simulink model "seti_ct"  (Simulink 6.2)
settings: Solver=ode45  StartTime=0.0  StopTime=100000  RelTol=1e-3
values from neighbouring files (symbols this model uses):
  bigColBits = 0    [address_gen_dram_mask.m]
  bigRowBits = log2(bigRowLength)    [address_gen_dram_mask.m]
  smallColBits = 0    [address_gen_dram_mask.m]
  smallRowBits = log2(smallRowLength)    [address_gen_dram_mask.m]
libraries: xbsIndex_r3 x487, xps_library x45, casper_library x18, fft_library x1
(part 2 of 3)

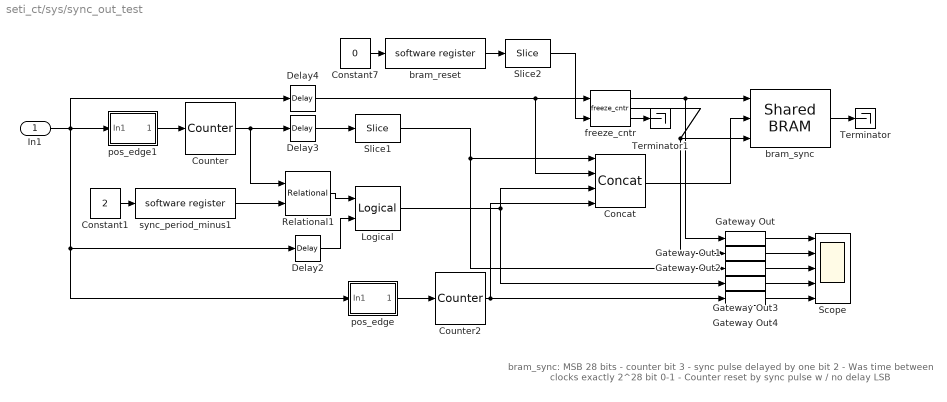
== system seti_ct/sys/sync_out_test ==
  note: bram_sync: MSB
      | 28 bits - counter
      | bit 3 - sync pulse delayed by one
      | bit 2 - Was time between clocks exactly 2^28
      | bit 0-1 - Counter reset by sync pulse w / no delay
      | LSB
  In1 : Inport  Port=1  LatchInput=off
  Concat : xbsIndex_r3/Concat  num_inputs=4  explicit_period=off  period=1  dbl_ovrd=off
  Constant1 : Constant  Value=2
  Constant7 : Constant  Value=0
  Counter : xbsIndex_r3/Counter  cnt_type=Free Running  n_bits=32  bin_pt=0  arith_type=Unsigned  start_count=0  cnt_to=2^4-1  cnt_by_val=1  operation=Up  explicit_period=on  period=1  load_pin=off  rst=on  en=off  dbl_ovrd=off  show_param=off  use_rpm=on  gen_core=off
      settings: xl_area=[0, 0, 0, 0, 0, 0, 0]
  Counter2 : xbsIndex_r3/Counter  cnt_type=Count Limited  n_bits=2  bin_pt=0  arith_type=Unsigned  start_count=0  cnt_to=3  cnt_by_val=1  operation=Up  explicit_period=on  period=1  load_pin=off  rst=on  en=off  dbl_ovrd=off  show_param=off  use_rpm=on  gen_core=off
      settings: xl_area=[0, 0, 0, 0, 0, 0, 0]
  Delay2 : xbsIndex_r3/Delay  latency=1  reg_retiming=off  explicit_period=on  period=1  en=off  accept_only_valid=off  init_zero=on  dbl_ovrd=off  show_param=off
      settings: xl_area=[0, 0, 0, 0, 0, 0, 0]
  Delay3 : xbsIndex_r3/Delay  latency=1  reg_retiming=off  explicit_period=on  period=1  en=off  accept_only_valid=off  init_zero=on  dbl_ovrd=off  show_param=off
      settings: xl_area=[0, 0, 0, 0, 0, 0, 0]
  Delay4 : xbsIndex_r3/Delay  latency=1  reg_retiming=off  explicit_period=on  period=1  en=off  accept_only_valid=off  init_zero=on  dbl_ovrd=off  show_param=off
      settings: xl_area=[0, 0, 0, 0, 0, 0, 0]
  Gateway Out{,1..4} (5 alike) : xbsIndex_r3/Gateway Out  output_type=Double  nbits=8  bin_pt=6  arith_type=Boolean  quantization=Truncate  overflow=Wrap  hdl_port=on  timing_constraint=None  locs_specified=off  LOCs={}  needs_fixed_name=off  show_param=off
      settings: xl_area=[0, 0, 0, 0, 0, 0, 0]
  Logical : xbsIndex_r3/Logical  logical_function=AND  inputs=2  precision=Full  arith_type=Unsigned  n_bits=2  bin_pt=0  align_bp=on  latency=0  explicit_period=off  period=1  en=off  dbl_ovrd=off  show_param=off
      settings: xl_area=[0, 0, 0, 0, 0, 0, 0]
  Relational1 : xbsIndex_r3/Relational  mode=a=b  latency=1  explicit_period=on  period=1  en=off  dbl_ovrd=off  show_param=off
      settings: xl_area=[0, 0, 0, 0, 0, 0, 0]
  Scope : Scope  NumInputPorts=5
      settings: YMin=-5~-5~-5~-5~-5  YMax=5~5~5~5~5
  Slice1 : xbsIndex_r3/Slice  mode=Lower Bit Location + Width  nbits=28  bit1=0  base1=MSB of Input  bit0=0  base0=LSB of Input  boolean_output=off  explicit_period=off  period=1  dbl_ovrd=off
  Slice2 : xbsIndex_r3/Slice  mode=Lower Bit Location + Width  nbits=1  bit1=0  base1=MSB of Input  bit0=0  base0=LSB of Input  boolean_output=on  explicit_period=off  period=1  dbl_ovrd=off
  Terminator : Terminator
  Terminator1 : Terminator
  bram_reset : xps_library/software register  Tag=xps:sw_reg  io_dir=From Processor  arith_type=Unsigned  bitwidth=32  bin_pt=0  sample_period=1  gw_name=seti_ct_sys_sync_out_test_bram_reset_user_data_out
  bram_sync : xps_library/Shared BRAM  Tag=xps:bram  arith_type=Unsigned  addr_width=12  data_width=32  data_bin_pt=0  init_vals=0  sample_rate=1
  freeze_cntr : casper_library/Misc/freeze_cntr  CounterBits=12
  pos_edge : Subsystem
  pos_edge1 : Subsystem
  sync_period_minus1 : xps_library/software register  Tag=xps:sw_reg  io_dir=From Processor  arith_type=Unsigned  bitwidth=32  bin_pt=0  sample_period=1  gw_name=seti_ct_sys_sync_out_test_sync_period_minus1_user_data_out
  wires:
  Counter/1 -> Relational1/1, Delay3/1
  Relational1/1 -> Logical/1
  Delay2/1 -> Logical/2
  Constant1/1 -> sync_period_minus1/1
  sync_period_minus1/1 -> Relational1/2
  freeze_cntr/1 -> bram_sync/1, Gateway Out/1
  freeze_cntr/2 -> bram_sync/3, Gateway Out1/1
  Delay3/1 -> Slice1/1
  Delay4/1 -> Concat/2, freeze_cntr/1
  Constant7/1 -> bram_reset/1
  bram_reset/1 -> Slice2/1
  Gateway Out/1 -> Scope/1
  Gateway Out1/1 -> Scope/2
  Gateway Out2/1 -> Scope/3
  Gateway Out3/1 -> Scope/4
  Concat/1 -> bram_sync/2
  Logical/1 -> Gateway Out3/1, Concat/3
  Slice2/1 -> freeze_cntr/2
  Gateway Out4/1 -> Scope/5
  pos_edge/1(Out1) -> Counter2/1
  Counter2/1 -> Gateway Out4/1, Concat/4
  pos_edge1/1(Out1) -> Counter/1
  Slice1/1 -> Concat/1, Gateway Out2/1
  In1/1 -> pos_edge1/1(In1), Delay4/1, Delay2/1, pos_edge/1(In1)
  bram_sync/1 -> Terminator/1
  freeze_cntr/3 -> Terminator1/1

== system seti_ct/sys/trig_delay ==
  data_in : Inport  Port=1  LatchInput=off
  trig_in : Inport  Port=2  LatchInput=off
  delay : Inport  Port=3  LatchInput=off
  Constant : xbsIndex_r3/Constant  const=1  equ=P=C  arith_type=Boolean  n_bits=32  bin_pt=0  opselect=C  inp2=PCIN>>17  opr=+  inp1=P  carry=CIN  iostate=0  explicit_period=on  period=1  dbl_ovrd=off
  Counter : xbsIndex_r3/Counter  cnt_type=Free Running  n_bits=32  bin_pt=0  arith_type=Unsigned  start_count=0  cnt_to=Inf  cnt_by_val=1  operation=Up  explicit_period=on  period=1  load_pin=off  rst=on  en=on  dbl_ovrd=off  show_param=off  use_rpm=on  gen_core=off
      settings: xl_area=[0, 0, 0, 0, 0, 0, 0]
  Delay : xbsIndex_r3/Delay  latency=2  reg_retiming=off  explicit_period=on  period=1  en=off  accept_only_valid=off  init_zero=on  dbl_ovrd=off  show_param=off
      settings: xl_area=[0, 0, 0, 0, 0, 0, 0]
  Gateway Out : xbsIndex_r3/Gateway Out  output_type=Double  nbits=8  bin_pt=6  arith_type=Boolean  quantization=Truncate  overflow=Wrap  hdl_port=on  timing_constraint=None  locs_specified=off  LOCs={}  needs_fixed_name=off  show_param=off
      settings: xl_area=[0, 0, 0, 0, 0, 0, 0]
  Gateway Out1 : xbsIndex_r3/Gateway Out  output_type=Double  nbits=8  bin_pt=6  arith_type=Boolean  quantization=Truncate  overflow=Wrap  hdl_port=on  timing_constraint=None  locs_specified=off  LOCs={}  needs_fixed_name=off  show_param=off
      settings: xl_area=[0, 0, 0, 0, 0, 0, 0]
  Register : xbsIndex_r3/Register  init=0  reg_only_valid=off  explicit_period=on  period=1  rst=on  en=on  out_en=off  dbl_ovrd=off  show_param=off
      settings: xl_area=[0, 0, 0, 0, 0, 0, 0]
  Relational : xbsIndex_r3/Relational  mode=a=b  latency=1  explicit_period=on  period=1  en=on  dbl_ovrd=off  show_param=off
      settings: xl_area=[0, 0, 0, 0, 0, 0, 0]
  Scope : Scope  NumInputPorts=2
      settings: YMin=-5~-5  YMax=5~5
  posedge : casper_library/Misc/posedge  Tag=Rising Edge Detector
  data_out : Outport
  trig_out : Outport  Port=2
  wires:
  delay/1 -> Relational/1
  trig_in/1 -> Register/3, Gateway Out1/1
  Constant/1 -> Register/1
  Relational/1 -> Register/2, Counter/1, Gateway Out/1, posedge/1
  Register/1 -> Counter/2, Relational/3
  Counter/1 -> Relational/2
  Gateway Out/1 -> Scope/1
  Gateway Out1/1 -> Scope/2
  data_in/1 -> Delay/1
  Delay/1 -> data_out/1
  posedge/1 -> trig_out/1

== system seti_ct/sys/trig_delay1 ==
  data_in : Inport  Port=1  LatchInput=off
  trig_in : Inport  Port=2  LatchInput=off
  delay : Inport  Port=3  LatchInput=off
  Constant : xbsIndex_r3/Constant  const=1  equ=P=C  arith_type=Boolean  n_bits=32  bin_pt=0  opselect=C  inp2=PCIN>>17  opr=+  inp1=P  carry=CIN  iostate=0  explicit_period=on  period=1  dbl_ovrd=off
  Counter : xbsIndex_r3/Counter  cnt_type=Free Running  n_bits=32  bin_pt=0  arith_type=Unsigned  start_count=0  cnt_to=Inf  cnt_by_val=1  operation=Up  explicit_period=on  period=1  load_pin=off  rst=on  en=on  dbl_ovrd=off  show_param=off  use_rpm=on  gen_core=off
      settings: xl_area=[0, 0, 0, 0, 0, 0, 0]
  Delay : xbsIndex_r3/Delay  latency=2  reg_retiming=off  explicit_period=on  period=1  en=off  accept_only_valid=off  init_zero=on  dbl_ovrd=off  show_param=off
      settings: xl_area=[0, 0, 0, 0, 0, 0, 0]
  Gateway Out : xbsIndex_r3/Gateway Out  output_type=Double  nbits=8  bin_pt=6  arith_type=Boolean  quantization=Truncate  overflow=Wrap  hdl_port=on  timing_constraint=None  locs_specified=off  LOCs={}  needs_fixed_name=off  show_param=off
      settings: xl_area=[0, 0, 0, 0, 0, 0, 0]
  Gateway Out1 : xbsIndex_r3/Gateway Out  output_type=Double  nbits=8  bin_pt=6  arith_type=Boolean  quantization=Truncate  overflow=Wrap  hdl_port=on  timing_constraint=None  locs_specified=off  LOCs={}  needs_fixed_name=off  show_param=off
      settings: xl_area=[0, 0, 0, 0, 0, 0, 0]
  Register : xbsIndex_r3/Register  init=0  reg_only_valid=off  explicit_period=on  period=1  rst=on  en=on  out_en=off  dbl_ovrd=off  show_param=off
      settings: xl_area=[0, 0, 0, 0, 0, 0, 0]
  Relational : xbsIndex_r3/Relational  mode=a=b  latency=1  explicit_period=on  period=1  en=on  dbl_ovrd=off  show_param=off
      settings: xl_area=[0, 0, 0, 0, 0, 0, 0]
  Scope : Scope  NumInputPorts=2
      settings: YMin=-5~-5  YMax=5~5
  posedge : casper_library/Misc/posedge  Tag=Rising Edge Detector
  data_out : Outport
  trig_out : Outport  Port=2
  wires:
  delay/1 -> Relational/1
  trig_in/1 -> Register/3, Gateway Out1/1
  Constant/1 -> Register/1
  Relational/1 -> Register/2, Counter/1, Gateway Out/1, posedge/1
  Register/1 -> Counter/2, Relational/3
  Counter/1 -> Relational/2
  Gateway Out/1 -> Scope/1
  Gateway Out1/1 -> Scope/2
  data_in/1 -> Delay/1
  Delay/1 -> data_out/1
  posedge/1 -> trig_out/1

== system seti_ct/sys/trig_delay2 ==
  data_in : Inport  Port=1  LatchInput=off
  trig_in : Inport  Port=2  LatchInput=off
  delay : Inport  Port=3  LatchInput=off
  Constant : xbsIndex_r3/Constant  const=1  equ=P=C  arith_type=Boolean  n_bits=32  bin_pt=0  opselect=C  inp2=PCIN>>17  opr=+  inp1=P  carry=CIN  iostate=0  explicit_period=on  period=1  dbl_ovrd=off
  Counter : xbsIndex_r3/Counter  cnt_type=Free Running  n_bits=32  bin_pt=0  arith_type=Unsigned  start_count=0  cnt_to=Inf  cnt_by_val=1  operation=Up  explicit_period=on  period=1  load_pin=off  rst=on  en=on  dbl_ovrd=off  show_param=off  use_rpm=on  gen_core=off
      settings: xl_area=[0, 0, 0, 0, 0, 0, 0]
  Delay : xbsIndex_r3/Delay  latency=2  reg_retiming=off  explicit_period=on  period=1  en=off  accept_only_valid=off  init_zero=on  dbl_ovrd=off  show_param=off
      settings: xl_area=[0, 0, 0, 0, 0, 0, 0]
  Gateway Out : xbsIndex_r3/Gateway Out  output_type=Double  nbits=8  bin_pt=6  arith_type=Boolean  quantization=Truncate  overflow=Wrap  hdl_port=on  timing_constraint=None  locs_specified=off  LOCs={}  needs_fixed_name=off  show_param=off
      settings: xl_area=[0, 0, 0, 0, 0, 0, 0]
  Gateway Out1 : xbsIndex_r3/Gateway Out  output_type=Double  nbits=8  bin_pt=6  arith_type=Boolean  quantization=Truncate  overflow=Wrap  hdl_port=on  timing_constraint=None  locs_specified=off  LOCs={}  needs_fixed_name=off  show_param=off
      settings: xl_area=[0, 0, 0, 0, 0, 0, 0]
  Register : xbsIndex_r3/Register  init=0  reg_only_valid=off  explicit_period=on  period=1  rst=on  en=on  out_en=off  dbl_ovrd=off  show_param=off
      settings: xl_area=[0, 0, 0, 0, 0, 0, 0]
  Relational : xbsIndex_r3/Relational  mode=a=b  latency=1  explicit_period=on  period=1  en=on  dbl_ovrd=off  show_param=off
      settings: xl_area=[0, 0, 0, 0, 0, 0, 0]
  Scope : Scope  NumInputPorts=2
      settings: YMin=-5~-5  YMax=5~5
  posedge : casper_library/Misc/posedge  Tag=Rising Edge Detector
  data_out : Outport
  trig_out : Outport  Port=2
  wires:
  delay/1 -> Relational/1
  trig_in/1 -> Register/3, Gateway Out1/1
  Constant/1 -> Register/1
  Relational/1 -> Register/2, Counter/1, Gateway Out/1, posedge/1
  Register/1 -> Counter/2, Relational/3
  Counter/1 -> Relational/2
  Gateway Out/1 -> Scope/1
  Gateway Out1/1 -> Scope/2
  data_in/1 -> Delay/1
  Delay/1 -> data_out/1
  posedge/1 -> trig_out/1

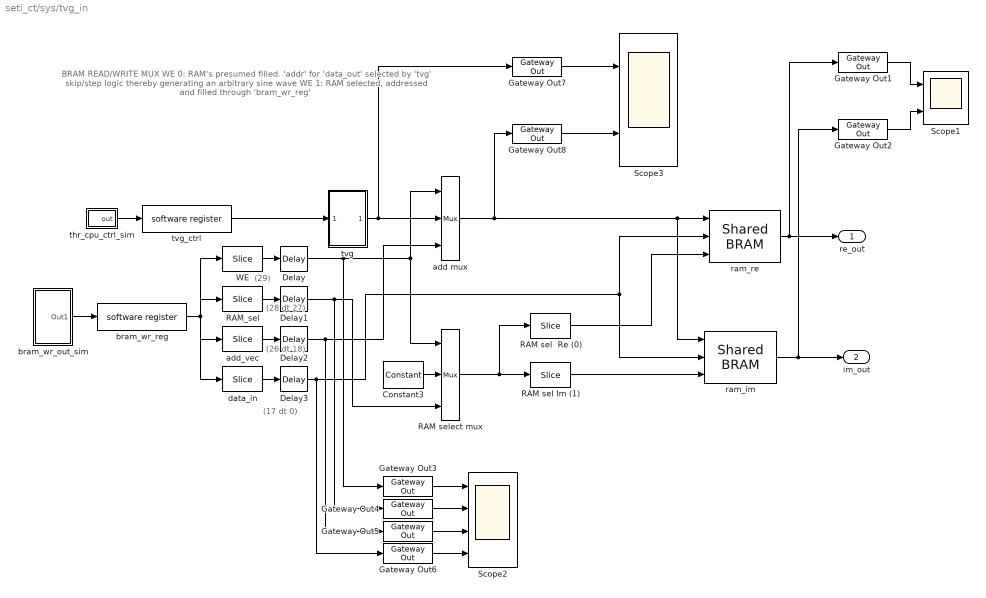
== system seti_ct/sys/tvg_in ==
  note: BRAM READ/WRITE MUX
      | WE 0: RAM's presumed filled.
      | 'addr' for 'data_out' selected
      | by 'tvg' skip/step logic thereby
      | generating an arbitrary sine wave
      | WE 1: RAM selected, addressed
      | and filled through
      | 'bram_wr_reg'
  note: (29)
  note: (28 dt 27)
  note: (17 dt 0)
  note: (26 dt 18)
  Constant3 : xbsIndex_r3/Constant  const=0  equ=P=C  arith_type=Unsigned  n_bits=4  bin_pt=0  opselect=C  inp2=PCIN>>17  opr=+  inp1=P  carry=CIN  iostate=0  explicit_period=on  period=1  dbl_ovrd=off
  Delay{,1..3} (4 alike) : xbsIndex_r3/Delay  latency=1  reg_retiming=off  explicit_period=on  period=1  en=off  accept_only_valid=off  init_zero=on  dbl_ovrd=off  show_param=off
      settings: xl_area=[0, 0, 0, 0, 0, 0, 0]
  Gateway Out{1..8} (8 alike) : xbsIndex_r3/Gateway Out  output_type=Double  nbits=8  bin_pt=6  arith_type=Boolean  quantization=Truncate  overflow=Wrap  hdl_port=on  timing_constraint=None  locs_specified=off  LOCs={}  needs_fixed_name=off  show_param=off
      settings: xl_area=[0, 0, 0, 0, 0, 0, 0]
  RAM sel  Re (0) : xbsIndex_r3/Slice  mode=Lower Bit Location + Width  nbits=1  bit1=0  base1=MSB of Input  bit0=0  base0=LSB of Input  boolean_output=on  explicit_period=on  period=1  dbl_ovrd=off
  RAM sel Im (1) : xbsIndex_r3/Slice  mode=Lower Bit Location + Width  nbits=1  bit1=0  base1=MSB of Input  bit0=1  base0=LSB of Input  boolean_output=on  explicit_period=on  period=1  dbl_ovrd=off
  RAM select mux : xbsIndex_r3/Mux  inputs=2  precision=Full  arith_type="Signed  (2's comp)"  n_bits=8  bin_pt=2  quantization=Truncate  overflow=Wrap  latency=0  explicit_period=on  period=1  en=off  dbl_ovrd=off  show_param=off  mux_type=off  use_rpm=off  gen_core=off
      settings: xl_area=[0, 0, 0, 0, 0, 0, 0]
  RAM_sel : xbsIndex_r3/Slice  mode=Lower Bit Location + Width  nbits=2  bit1=10  base1=MSB of Input  bit0=27  base0=LSB of Input  boolean_output=off  explicit_period=on  period=1  dbl_ovrd=off
  Scope1 : Scope  NumInputPorts=2
      settings: YMin=-5~-5  YMax=5~5  SaveName=ScopeData2
  Scope2 : Scope  NumInputPorts=4
      settings: YMin=-5~-5~-5~-5  YMax=5~5~5~5
  Scope3 : Scope  NumInputPorts=2
      settings: YMin=-5~-5  YMax=5~5  SaveName=ScopeData3
  WE : xbsIndex_r3/Slice  mode=Lower Bit Location + Width  nbits=1  bit1=10  base1=MSB of Input  bit0=29  base0=LSB of Input  boolean_output=off  explicit_period=on  period=1  dbl_ovrd=off
  add mux : xbsIndex_r3/Mux  inputs=2  precision=Full  arith_type="Signed  (2's comp)"  n_bits=8  bin_pt=2  quantization=Truncate  overflow=Wrap  latency=0  explicit_period=on  period=1  en=off  dbl_ovrd=off  show_param=off  mux_type=off  use_rpm=off  gen_core=off
      settings: xl_area=[0, 0, 0, 0, 0, 0, 0]
  add_vec : xbsIndex_r3/Slice  mode=Lower Bit Location + Width  nbits=9  bit1=0  base1=MSB of Input  bit0=18  base0=LSB of Input  boolean_output=off  explicit_period=on  period=1  dbl_ovrd=off
  bram_wr_out_sim : Subsystem  mask{we_enable=0, ram_sel=3, add_vec=512, data_in=32}
      mask prompts: we_enable "Write enable"; ram_sel "RAM selector (1 = Re; 2 = Im; 3 = both)"; add_vec "RAM address"; data_in "Data in"
  bram_wr_reg : xps_library/software register  Tag=xps:sw_reg  io_dir=From Processor  arith_type=Unsigned  bitwidth=32  bin_pt=0  sample_period=1  gw_name=seti_ct_sys_tvg_in_bram_wr_reg_user_data_out
  data_in : xbsIndex_r3/Slice  mode=Lower Bit Location + Width  nbits=18  bit1=0  base1=MSB of Input  bit0=0  base0=LSB of Input  boolean_output=off  explicit_period=on  period=1  dbl_ovrd=off
  ram_im : xps_library/Shared BRAM  Tag=xps:bram  arith_type="Signed  (2's comp)"  addr_width=11  data_width=32  data_bin_pt=0  init_vals=[1:2^11]  sample_rate=1
  ram_re : xps_library/Shared BRAM  Tag=xps:bram  arith_type="Signed  (2's comp)"  addr_width=11  data_width=32  data_bin_pt=0  init_vals=[1:2^11]  sample_rate=1
  thr_cpu_ctrl_sim : Subsystem  mask{tvg_skip=1, tvg_stall=2, tvg_length=5}
      mask prompts: tvg_skip "Skip"; tvg_stall "Stall"; tvg_length "Length"
      mask help:
      | Mux Data for CT and FFT Syncs:
      |
      | 0 -> Interchip Connection
      | 1 -> User Generated External Sync
      | 2 -> Periodic Sync Generator
      | 3 -> Periodic Sync Generator (Same as 2)
      |
      | Mux Data for CT and FFT Inputs:
      |
      | 0 -> Interchip Connection
      | 1 -> Test Vector Generator (TVG)
      | 2 -> All Zeroes (0's)
      | 3 -> All Ones (1's)
  tvg : Subsystem  mask(Test Vector Generator(TVG)){tvg_skip=1, tvg_stall=1, tvg_length=512}
      mask prompts: tvg_skip "Skip"; tvg_stall "Stall"; tvg_length "Length"
  tvg_ctrl : xps_library/software register  Tag=xps:sw_reg  io_dir=From Processor  arith_type=Unsigned  bitwidth=32  bin_pt=0  sample_period=1  gw_name=seti_ct_sys_tvg_in_tvg_ctrl_user_data_out
  re_out : Outport
  im_out : Outport  Port=2
  wires:
  tvg_ctrl/1 -> tvg/1(In1)
  tvg/1(Out1) -> add mux/2, Gateway Out7/1
  Constant3/1 -> RAM select mux/2
  RAM select mux/1 -> RAM sel  Re (0)/1, RAM sel Im (1)/1
  RAM sel  Re (0)/1 -> ram_re/3
  WE/1 -> Delay/1
  Gateway Out1/1 -> Scope1/1
  Gateway Out2/1 -> Scope1/2
  thr_cpu_ctrl_sim/1(out) -> tvg_ctrl/1
  bram_wr_reg/1 -> data_in/1, add_vec/1, RAM_sel/1, WE/1
  add_vec/1 -> Delay2/1
  RAM_sel/1 -> Delay1/1
  add mux/1 -> ram_im/1, ram_re/1, Gateway Out8/1
  data_in/1 -> Delay3/1
  RAM sel Im (1)/1 -> ram_im/3
  ram_re/1 -> Gateway Out1/1, re_out/1
  ram_im/1 -> Gateway Out2/1, im_out/1
  bram_wr_out_sim/1(Out1) -> bram_wr_reg/1
  Gateway Out3/1 -> Scope2/1
  Gateway Out4/1 -> Scope2/2
  Gateway Out5/1 -> Scope2/3
  Gateway Out6/1 -> Scope2/4
  Delay/1 -> Gateway Out3/1, add mux/1, RAM select mux/1
  Delay1/1 -> Gateway Out4/1, RAM select mux/3
  Delay2/1 -> Gateway Out5/1, add mux/3
  Delay3/1 -> Gateway Out6/1, ram_re/2, ram_im/2
  Gateway Out7/1 -> Scope3/1
  Gateway Out8/1 -> Scope3/2

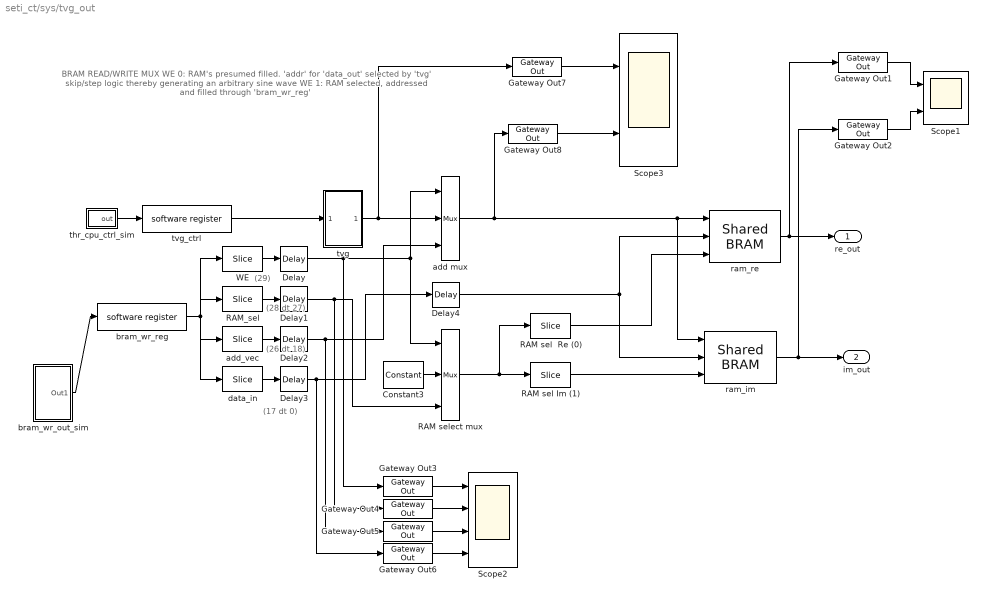
== system seti_ct/sys/tvg_out ==
  note: BRAM READ/WRITE MUX
      | WE 0: RAM's presumed filled.
      | 'addr' for 'data_out' selected
      | by 'tvg' skip/step logic thereby
      | generating an arbitrary sine wave
      | WE 1: RAM selected, addressed
      | and filled through
      | 'bram_wr_reg'
  note: (29)
  note: (28 dt 27)
  note: (17 dt 0)
  note: (26 dt 18)
  Constant3 : xbsIndex_r3/Constant  const=0  equ=P=C  arith_type=Unsigned  n_bits=4  bin_pt=0  opselect=C  inp2=PCIN>>17  opr=+  inp1=P  carry=CIN  iostate=0  explicit_period=on  period=1  dbl_ovrd=off
  Delay{,1..4} (5 alike) : xbsIndex_r3/Delay  latency=1  reg_retiming=off  explicit_period=on  period=1  en=off  accept_only_valid=off  init_zero=on  dbl_ovrd=off  show_param=off
      settings: xl_area=[0, 0, 0, 0, 0, 0, 0]
  Gateway Out{1..8} (8 alike) : xbsIndex_r3/Gateway Out  output_type=Double  nbits=8  bin_pt=6  arith_type=Boolean  quantization=Truncate  overflow=Wrap  hdl_port=on  timing_constraint=None  locs_specified=off  LOCs={}  needs_fixed_name=off  show_param=off
      settings: xl_area=[0, 0, 0, 0, 0, 0, 0]
  RAM sel  Re (0) : xbsIndex_r3/Slice  mode=Lower Bit Location + Width  nbits=1  bit1=0  base1=MSB of Input  bit0=0  base0=LSB of Input  boolean_output=on  explicit_period=on  period=1  dbl_ovrd=off
  RAM sel Im (1) : xbsIndex_r3/Slice  mode=Lower Bit Location + Width  nbits=1  bit1=0  base1=MSB of Input  bit0=1  base0=LSB of Input  boolean_output=on  explicit_period=on  period=1  dbl_ovrd=off
  RAM select mux : xbsIndex_r3/Mux  inputs=2  precision=Full  arith_type="Signed  (2's comp)"  n_bits=8  bin_pt=2  quantization=Truncate  overflow=Wrap  latency=1  explicit_period=on  period=1  en=off  dbl_ovrd=off  show_param=off  mux_type=off  use_rpm=off  gen_core=off
      settings: xl_area=[0, 0, 0, 0, 0, 0, 0]
  RAM_sel : xbsIndex_r3/Slice  mode=Lower Bit Location + Width  nbits=2  bit1=10  base1=MSB of Input  bit0=27  base0=LSB of Input  boolean_output=off  explicit_period=on  period=1  dbl_ovrd=off
  Scope1 : Scope  NumInputPorts=2
      settings: YMin=-5~-5  YMax=5~5  SaveName=ScopeData2
  Scope2 : Scope  NumInputPorts=4
      settings: YMin=-5~-5~-5~-5  YMax=5~5~5~5
  Scope3 : Scope  NumInputPorts=2
      settings: YMin=-5~-5  YMax=5~5  SaveName=ScopeData3
  WE : xbsIndex_r3/Slice  mode=Lower Bit Location + Width  nbits=1  bit1=10  base1=MSB of Input  bit0=29  base0=LSB of Input  boolean_output=off  explicit_period=on  period=1  dbl_ovrd=off
  add mux : xbsIndex_r3/Mux  inputs=2  precision=Full  arith_type="Signed  (2's comp)"  n_bits=8  bin_pt=2  quantization=Truncate  overflow=Wrap  latency=1  explicit_period=on  period=1  en=off  dbl_ovrd=off  show_param=off  mux_type=off  use_rpm=off  gen_core=off
      settings: xl_area=[0, 0, 0, 0, 0, 0, 0]
  add_vec : xbsIndex_r3/Slice  mode=Lower Bit Location + Width  nbits=9  bit1=0  base1=MSB of Input  bit0=18  base0=LSB of Input  boolean_output=off  explicit_period=on  period=1  dbl_ovrd=off
  bram_wr_out_sim : Subsystem  mask{we_enable=0, ram_sel=3, add_vec=512, data_in=32}
      mask prompts: we_enable "Write enable"; ram_sel "RAM selector (1 = Re; 2 = Im; 3 = both)"; add_vec "RAM address"; data_in "Data in"
  bram_wr_reg : xps_library/software register  Tag=xps:sw_reg  io_dir=From Processor  arith_type=Unsigned  bitwidth=32  bin_pt=0  sample_period=1  gw_name=seti_ct_sys_tvg_out_bram_wr_reg_user_data_out
  data_in : xbsIndex_r3/Slice  mode=Lower Bit Location + Width  nbits=18  bit1=0  base1=MSB of Input  bit0=0  base0=LSB of Input  boolean_output=off  explicit_period=on  period=1  dbl_ovrd=off
  ram_im : xps_library/Shared BRAM  Tag=xps:bram  arith_type="Signed  (2's comp)"  addr_width=11  data_width=32  data_bin_pt=0  init_vals=[1:2^11]  sample_rate=1
  ram_re : xps_library/Shared BRAM  Tag=xps:bram  arith_type="Signed  (2's comp)"  addr_width=11  data_width=32  data_bin_pt=0  init_vals=[1:2^11]  sample_rate=1
  thr_cpu_ctrl_sim : Subsystem  mask{tvg_skip=1, tvg_stall=2, tvg_length=5}
      mask prompts: tvg_skip "Skip"; tvg_stall "Stall"; tvg_length "Length"
      mask help:
      | Mux Data for CT and FFT Syncs:
      |
      | 0 -> Interchip Connection
      | 1 -> User Generated External Sync
      | 2 -> Periodic Sync Generator
      | 3 -> Periodic Sync Generator (Same as 2)
      |
      | Mux Data for CT and FFT Inputs:
      |
      | 0 -> Interchip Connection
      | 1 -> Test Vector Generator (TVG)
      | 2 -> All Zeroes (0's)
      | 3 -> All Ones (1's)
  tvg : Subsystem  mask(Test Vector Generator(TVG)){tvg_skip=1, tvg_stall=1, tvg_length=512}
      mask prompts: tvg_skip "Skip"; tvg_stall "Stall"; tvg_length "Length"
  tvg_ctrl : xps_library/software register  Tag=xps:sw_reg  io_dir=From Processor  arith_type=Unsigned  bitwidth=32  bin_pt=0  sample_period=1  gw_name=seti_ct_sys_tvg_out_tvg_ctrl_user_data_out
  re_out : Outport
  im_out : Outport  Port=2
  wires:
  tvg_ctrl/1 -> tvg/1(In1)
  tvg/1(Out1) -> add mux/2, Gateway Out7/1
  Constant3/1 -> RAM select mux/2
  RAM select mux/1 -> RAM sel  Re (0)/1, RAM sel Im (1)/1
  RAM sel  Re (0)/1 -> ram_re/3
  WE/1 -> Delay/1
  Gateway Out1/1 -> Scope1/1
  Gateway Out2/1 -> Scope1/2
  thr_cpu_ctrl_sim/1(out) -> tvg_ctrl/1
  bram_wr_reg/1 -> data_in/1, add_vec/1, RAM_sel/1, WE/1
  add_vec/1 -> Delay2/1
  RAM_sel/1 -> Delay1/1
  add mux/1 -> ram_im/1, ram_re/1, Gateway Out8/1
  data_in/1 -> Delay3/1
  RAM sel Im (1)/1 -> ram_im/3
  ram_re/1 -> Gateway Out1/1, re_out/1
  ram_im/1 -> Gateway Out2/1, im_out/1
  bram_wr_out_sim/1(Out1) -> bram_wr_reg/1
  Gateway Out3/1 -> Scope2/1
  Gateway Out4/1 -> Scope2/2
  Gateway Out5/1 -> Scope2/3
  Gateway Out6/1 -> Scope2/4
  Delay/1 -> Gateway Out3/1, add mux/1, RAM select mux/1
  Delay1/1 -> Gateway Out4/1, RAM select mux/3
  Delay2/1 -> Gateway Out5/1, add mux/3
  Delay3/1 -> Gateway Out6/1, Delay4/1
  Gateway Out7/1 -> Scope3/1
  Gateway Out8/1 -> Scope3/2
  Delay4/1 -> ram_re/2, ram_im/2

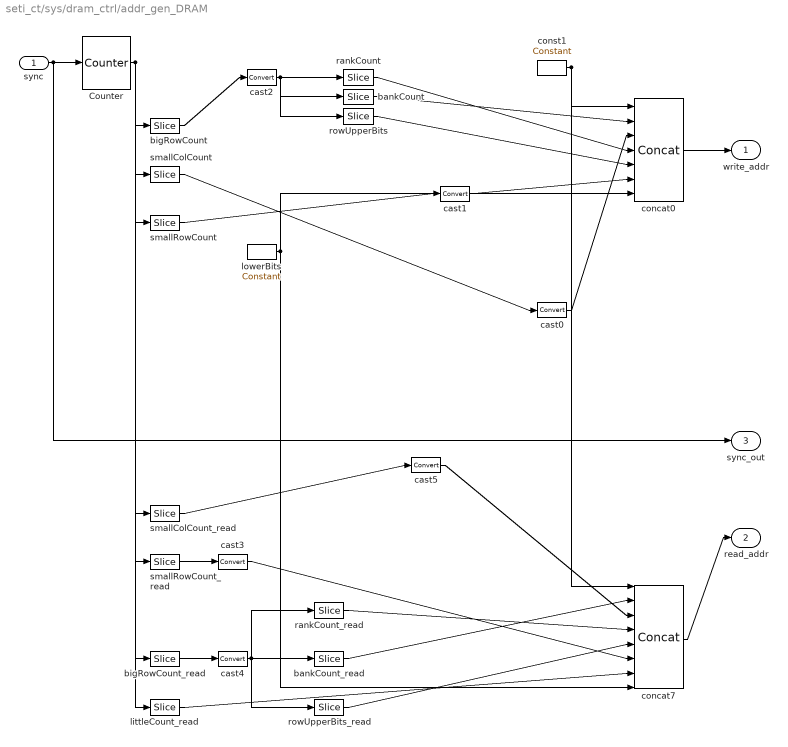
== system seti_ct/sys/dram_ctrl/addr_gen_DRAM ==
  sync : Inport  Port=1  LatchInput=off
  Counter : xbsIndex_r3/Counter  cnt_type=Free Running  n_bits=counterBitwidth  bin_pt=0  arith_type=Unsigned  start_count=0  cnt_to=Inf  cnt_by_val=1  operation=Up  explicit_period=off  period=1  load_pin=off  rst=on  en=off  dbl_ovrd=off  show_param=off  use_rpm=on  gen_core=off
      settings: xl_area=[0, 0, 0, 0, 0, 0, 0]
  bankCount : xbsIndex_r3/Slice  mode=Upper Bit Location + Width  nbits=2  bit1=-1  base1=MSB of Input  bit0=0  base0=LSB of Input  boolean_output=off  explicit_period=off  period=1  dbl_ovrd=off
  bankCount_read : xbsIndex_r3/Slice  mode=Upper Bit Location + Width  nbits=2  bit1=-1  base1=MSB of Input  bit0=0  base0=LSB of Input  boolean_output=off  explicit_period=off  period=1  dbl_ovrd=off
  bigRowCount : xbsIndex_r3/Slice  mode=Lower Bit Location + Width  nbits=bigRowBits  bit1=0  base1=MSB of Input  bit0=smallRowBits+smallColBits  base0=LSB of Input  boolean_output=off  explicit_period=off  period=1  dbl_ovrd=off
  bigRowCount_read : xbsIndex_r3/Slice  mode=Lower Bit Location + Width  nbits=bigRowBits  bit1=0  base1=MSB of Input  bit0=2  base0=LSB of Input  boolean_output=off  explicit_period=off  period=1  dbl_ovrd=off
  cast0 : xbsIndex_r3/Convert  arith_type=Unsigned  n_bits=14  bin_pt=0  quantization=Truncate  overflow=Wrap  latency=0  explicit_period=off  period=1  dbl_ovrd=off  show_param=off  inserted_by_tool=off  pipeline=off
      settings: xl_area=[0, 0, 0, 0, 0, 0, 0]
  cast1 : xbsIndex_r3/Convert  arith_type=Unsigned  n_bits=6  bin_pt=0  quantization=Truncate  overflow=Wrap  latency=0  explicit_period=off  period=1  dbl_ovrd=off  show_param=off  inserted_by_tool=off  pipeline=off
      settings: xl_area=[0, 0, 0, 0, 0, 0, 0]
  cast2 : xbsIndex_r3/Convert  arith_type=Unsigned  n_bits=7  bin_pt=0  quantization=Truncate  overflow=Wrap  latency=0  explicit_period=off  period=1  dbl_ovrd=off  show_param=off  inserted_by_tool=off  pipeline=off
      settings: xl_area=[0, 0, 0, 0, 0, 0, 0]
  cast3 : xbsIndex_r3/Convert  arith_type=Unsigned  n_bits=4  bin_pt=0  quantization=Truncate  overflow=Wrap  latency=0  explicit_period=off  period=1  dbl_ovrd=off  show_param=off  inserted_by_tool=off  pipeline=off
      settings: xl_area=[0, 0, 0, 0, 0, 0, 0]
  cast4 : xbsIndex_r3/Convert  arith_type=Unsigned  n_bits=7  bin_pt=0  quantization=Truncate  overflow=Wrap  latency=0  explicit_period=off  period=1  dbl_ovrd=off  show_param=off  inserted_by_tool=off  pipeline=off
      settings: xl_area=[0, 0, 0, 0, 0, 0, 0]
  cast5 : xbsIndex_r3/Convert  arith_type=Unsigned  n_bits=14  bin_pt=0  quantization=Truncate  overflow=Wrap  latency=0  explicit_period=off  period=1  dbl_ovrd=off  show_param=off  inserted_by_tool=off  pipeline=off
      settings: xl_area=[0, 0, 0, 0, 0, 0, 0]
  concat0 : xbsIndex_r3/Concat  num_inputs=7  explicit_period=off  period=1  dbl_ovrd=off
  concat7 : xbsIndex_r3/Concat  num_inputs=8  explicit_period=off  period=1  dbl_ovrd=off
  const1 : xbsIndex_r3/Constant  const=0  equ=P=C  arith_type=Unsigned  n_bits=2  bin_pt=0  opselect=C  inp2=PCIN>>17  opr=+  inp1=P  carry=CIN  iostate=0  explicit_period=on  period=1  dbl_ovrd=off
  littleCount_read : xbsIndex_r3/Slice  mode=Lower Bit Location + Width  nbits=2  bit1=0  base1=MSB of Input  bit0=0  base0=LSB of Input  boolean_output=off  explicit_period=off  period=1  dbl_ovrd=off
  lowerBits : xbsIndex_r3/Constant  const=0  equ=P=C  arith_type=Unsigned  n_bits=3  bin_pt=0  opselect=C  inp2=PCIN>>17  opr=+  inp1=P  carry=CIN  iostate=0  explicit_period=on  period=1  dbl_ovrd=off
  rankCount : xbsIndex_r3/Slice  mode=Upper Bit Location + Width  nbits=1  bit1=0  base1=MSB of Input  bit0=0  base0=LSB of Input  boolean_output=off  explicit_period=off  period=1  dbl_ovrd=off
  rankCount_read : xbsIndex_r3/Slice  mode=Upper Bit Location + Width  nbits=1  bit1=0  base1=MSB of Input  bit0=0  base0=LSB of Input  boolean_output=off  explicit_period=off  period=1  dbl_ovrd=off
  rowUpperBits : xbsIndex_r3/Slice  mode=Lower Bit Location + Width  nbits=4  bit1=0  base1=MSB of Input  bit0=0  base0=LSB of Input  boolean_output=off  explicit_period=off  period=1  dbl_ovrd=off
  rowUpperBits_read : xbsIndex_r3/Slice  mode=Lower Bit Location + Width  nbits=4  bit1=0  base1=MSB of Input  bit0=0  base0=LSB of Input  boolean_output=off  explicit_period=off  period=1  dbl_ovrd=off
  smallColCount : xbsIndex_r3/Slice  mode=Lower Bit Location + Width  nbits=smallColBits  bit1=0  base1=MSB of Input  bit0=smallRowBits  base0=LSB of Input  boolean_output=off  explicit_period=off  period=1  dbl_ovrd=off
  smallColCount_read : xbsIndex_r3/Slice  mode=Lower Bit Location + Width  nbits=smallColBits  bit1=0  base1=MSB of Input  bit0=bigRowBits+bigColBits+smallRowBits  base0=LSB of Input  boolean_output=off  explicit_period=off  period=1  dbl_ovrd=off
  smallRowCount : xbsIndex_r3/Slice  mode=Lower Bit Location + Width  nbits=smallRowBits  bit1=0  base1=MSB of Input  bit0=0  base0=LSB of Input  boolean_output=off  explicit_period=off  period=1  dbl_ovrd=off
  smallRowCount_read : xbsIndex_r3/Slice  mode=Lower Bit Location + Width  nbits=smallRowBits-2  bit1=0  base1=MSB of Input  bit0=bigRowBits+bigColBits+2  base0=LSB of Input  boolean_output=off  explicit_period=off  period=1  dbl_ovrd=off
  write_addr : Outport
  read_addr : Outport  Port=2
  sync_out : Outport  Port=3
  wires:
  Counter/1 -> smallColCount/1, smallColCount_read/1, smallRowCount/1, bigRowCount/1, smallRowCount_read/1, bigRowCount_read/1, littleCount_read/1
  smallColCount/1 -> cast0/1
  smallColCount_read/1 -> cast5/1
  sync/1 -> Counter/1, sync_out/1
  lowerBits/1 -> concat0/7, concat7/8
  cast0/1 -> concat0/3
  cast1/1 -> concat0/6
  rankCount/1 -> concat0/4
  smallRowCount/1 -> cast1/1
  rowUpperBits/1 -> concat0/5
  bankCount/1 -> concat0/2
  const1/1 -> concat0/1, concat7/1
  bigRowCount/1 -> cast2/1
  cast2/1 -> bankCount/1, rankCount/1, rowUpperBits/1
  concat0/1 -> write_addr/1
  smallRowCount_read/1 -> cast3/1
  bigRowCount_read/1 -> cast4/1
  cast4/1 -> rankCount_read/1, bankCount_read/1, rowUpperBits_read/1
  concat7/1 -> read_addr/1
  bankCount_read/1 -> concat7/2
  cast5/1 -> concat7/3
  rankCount_read/1 -> concat7/4
  rowUpperBits_read/1 -> concat7/5
  cast3/1 -> concat7/6
  littleCount_read/1 -> concat7/7

== system seti_ct/sys/dram_ctrl/cmdAck1 ==
  in : Inport  Port=1  LatchInput=off
  Scope : Scope
  big_negedge : Subsystem
  gpio : xps_library/gpio  Tag=xps:gpio  io_group=BEE2_usr:led  io_dir=out  arith_type=Unsigned  bitwidth=1  bin_pt=0  bit_index=1  sample_period=1  use_single_ended=off  use_ddr=off  reg_iob=on  reg_clk_phase=0  termination=None
  wires:
  gpio/1 -> Scope/1
  in/1 -> big_negedge/1(in)
  big_negedge/1(pulse) -> gpio/1

== system seti_ct/sys/dram_ctrl/cmdAck2 ==
  in : Inport  Port=1  LatchInput=off
  Scope : Scope
  big_negedge : Subsystem
  gpio : xps_library/gpio  Tag=xps:gpio  io_group=BEE2_usr:led  io_dir=out  arith_type=Unsigned  bitwidth=1  bin_pt=0  bit_index=2  sample_period=1  use_single_ended=off  use_ddr=off  reg_iob=off  reg_clk_phase=0  termination=None
  wires:
  in/1 -> big_negedge/1(in)
  big_negedge/1(pulse) -> gpio/1
  gpio/1 -> Scope/1

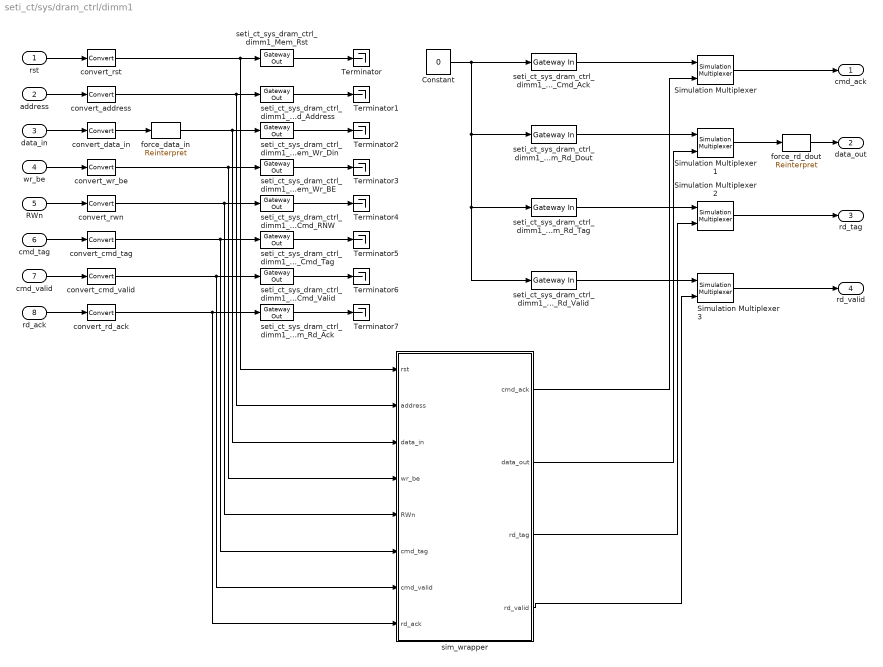
== system seti_ct/sys/dram_ctrl/dimm1 ==
  rst : Inport  Port=1  LatchInput=off
  address : Inport  Port=2  LatchInput=off
  data_in : Inport  Port=3  LatchInput=off
  wr_be : Inport  Port=4  LatchInput=off
  RWn : Inport  Port=5  LatchInput=off
  cmd_tag : Inport  Port=6  LatchInput=off
  cmd_valid : Inport  Port=7  LatchInput=off
  rd_ack : Inport  Port=8  LatchInput=off
  Constant : Constant  Value=0
  Simulation Multiplexer{,1..3} (4 alike) : xbsIndex_r3/Simulation Multiplexer  sim_sel=2  hw_sel=1
  Terminator{,1..7} (8 alike) : Terminator
  convert_address : xbsIndex_r3/Convert  arith_type=Unsigned  n_bits=32  bin_pt=0  quantization=Truncate  overflow=Wrap  latency=0  explicit_period=off  period=sample_period  dbl_ovrd=off  show_param=off  inserted_by_tool=off  pipeline=off
      settings: xl_area=[0, 0, 0, 0, 0, 0, 0]
  convert_cmd_tag : xbsIndex_r3/Convert  arith_type=Unsigned  n_bits=32  bin_pt=0  quantization=Truncate  overflow=Wrap  latency=0  explicit_period=off  period=1  dbl_ovrd=off  show_param=off  inserted_by_tool=off  pipeline=off
      settings: xl_area=[0, 0, 0, 0, 0, 0, 0]
  convert_cmd_valid : xbsIndex_r3/Convert  arith_type=Unsigned  n_bits=1  bin_pt=0  quantization=Truncate  overflow=Wrap  latency=0  explicit_period=off  period=1  dbl_ovrd=off  show_param=off  inserted_by_tool=off  pipeline=off
      settings: xl_area=[0, 0, 0, 0, 0, 0, 0]
  convert_data_in : xbsIndex_r3/Convert  arith_type=Unsigned  n_bits=144  bin_pt=0  quantization=Truncate  overflow=Wrap  latency=0  explicit_period=off  period=sample_period  dbl_ovrd=off  show_param=off  inserted_by_tool=off  pipeline=off
      settings: xl_area=[0, 0, 0, 0, 0, 0, 0]
  convert_rd_ack : xbsIndex_r3/Convert  arith_type=Unsigned  n_bits=1  bin_pt=0  quantization=Truncate  overflow=Wrap  latency=0  explicit_period=off  period=1  dbl_ovrd=off  show_param=off  inserted_by_tool=off  pipeline=off
      settings: xl_area=[0, 0, 0, 0, 0, 0, 0]
  convert_rst : xbsIndex_r3/Convert  arith_type=Unsigned  n_bits=1  bin_pt=0  quantization=Truncate  overflow=Wrap  latency=0  explicit_period=off  period=sample_period  dbl_ovrd=off  show_param=off  inserted_by_tool=off  pipeline=off
      settings: xl_area=[0, 0, 0, 0, 0, 0, 0]
  convert_rwn : xbsIndex_r3/Convert  arith_type=Unsigned  n_bits=1  bin_pt=0  quantization=Truncate  overflow=Wrap  latency=0  explicit_period=off  period=1  dbl_ovrd=off  show_param=off  inserted_by_tool=off  pipeline=off
      settings: xl_area=[0, 0, 0, 0, 0, 0, 0]
  convert_wr_be : xbsIndex_r3/Convert  arith_type=Unsigned  n_bits=18  bin_pt=0  quantization=Truncate  overflow=Wrap  latency=0  explicit_period=off  period=1  dbl_ovrd=off  show_param=off  inserted_by_tool=off  pipeline=off
      settings: xl_area=[0, 0, 0, 0, 0, 0, 0]
  force_data_in : xbsIndex_r3/Reinterpret  force_arith_type=on  arith_type=Unsigned  force_bin_pt=on  bin_pt=0  force_valid=on
  force_rd_dout : xbsIndex_r3/Reinterpret  force_arith_type=on  arith_type=Unsigned  force_bin_pt=on  bin_pt=0  force_valid=on
  seti_ct_sys_dram_ctrl_dimm1_Mem_Cmd_Ack : xbsIndex_r3/Gateway In  arith_type=Unsigned  n_bits=1  bin_pt=0  quantization=Truncate  overflow=Wrap  period=sample_period  timing_constraint=None  locs_specified=off  LOCs={}  needs_fixed_name=off  dbl_ovrd=off  show_param=off
      settings: xl_area=[0, 0, 0, 0, 0, 0, 0]
  seti_ct_sys_dram_ctrl_dimm1_Mem_Cmd_Address : xbsIndex_r3/Gateway Out  output_type=Double  nbits=8  bin_pt=6  arith_type=Boolean  quantization=Truncate  overflow=Wrap  hdl_port=on  timing_constraint=None  locs_specified=off  LOCs={}  needs_fixed_name=off  show_param=off
      settings: xl_area=[0, 0, 0, 0, 0, 0, 0]
  seti_ct_sys_dram_ctrl_dimm1_Mem_Cmd_RNW : xbsIndex_r3/Gateway Out  output_type=Double  nbits=8  bin_pt=6  arith_type=Boolean  quantization=Truncate  overflow=Wrap  hdl_port=on  timing_constraint=None  locs_specified=off  LOCs={}  needs_fixed_name=off  show_param=off
      settings: xl_area=[0, 0, 0, 0, 0, 0, 0]
  seti_ct_sys_dram_ctrl_dimm1_Mem_Cmd_Tag : xbsIndex_r3/Gateway Out  output_type=Double  nbits=8  bin_pt=6  arith_type=Boolean  quantization=Truncate  overflow=Wrap  hdl_port=on  timing_constraint=None  locs_specified=off  LOCs={}  needs_fixed_name=off  show_param=off
      settings: xl_area=[0, 0, 0, 0, 0, 0, 0]
  seti_ct_sys_dram_ctrl_dimm1_Mem_Cmd_Valid : xbsIndex_r3/Gateway Out  output_type=Double  nbits=8  bin_pt=6  arith_type=Boolean  quantization=Truncate  overflow=Wrap  hdl_port=on  timing_constraint=None  locs_specified=off  LOCs={}  needs_fixed_name=off  show_param=off
      settings: xl_area=[0, 0, 0, 0, 0, 0, 0]
  seti_ct_sys_dram_ctrl_dimm1_Mem_Rd_Ack : xbsIndex_r3/Gateway Out  output_type=Double  nbits=8  bin_pt=6  arith_type=Boolean  quantization=Truncate  overflow=Wrap  hdl_port=on  timing_constraint=None  locs_specified=off  LOCs={}  needs_fixed_name=off  show_param=off
      settings: xl_area=[0, 0, 0, 0, 0, 0, 0]
  seti_ct_sys_dram_ctrl_dimm1_Mem_Rd_Dout : xbsIndex_r3/Gateway In  arith_type=Unsigned  n_bits=144  bin_pt=0  quantization=Truncate  overflow=Wrap  period=sample_period  timing_constraint=None  locs_specified=off  LOCs={}  needs_fixed_name=off  dbl_ovrd=off  show_param=off
      settings: xl_area=[0, 0, 0, 0, 0, 0, 0]
  seti_ct_sys_dram_ctrl_dimm1_Mem_Rd_Tag : xbsIndex_r3/Gateway In  arith_type=Unsigned  n_bits=32  bin_pt=0  quantization=Truncate  overflow=Wrap  period=sample_period  timing_constraint=None  locs_specified=off  LOCs={}  needs_fixed_name=off  dbl_ovrd=off  show_param=off
      settings: xl_area=[0, 0, 0, 0, 0, 0, 0]
  seti_ct_sys_dram_ctrl_dimm1_Mem_Rd_Valid : xbsIndex_r3/Gateway In  arith_type=Unsigned  n_bits=1  bin_pt=0  quantization=Truncate  overflow=Wrap  period=sample_period  timing_constraint=None  locs_specified=off  LOCs={}  needs_fixed_name=off  dbl_ovrd=off  show_param=off
      settings: xl_area=[0, 0, 0, 0, 0, 0, 0]
  seti_ct_sys_dram_ctrl_dimm1_Mem_Rst : xbsIndex_r3/Gateway Out  output_type=Double  nbits=8  bin_pt=6  arith_type=Boolean  quantization=Truncate  overflow=Wrap  hdl_port=on  timing_constraint=None  locs_specified=off  LOCs={}  needs_fixed_name=off  show_param=off
      settings: xl_area=[0, 0, 0, 0, 0, 0, 0]
  seti_ct_sys_dram_ctrl_dimm1_Mem_Wr_BE : xbsIndex_r3/Gateway Out  output_type=Double  nbits=8  bin_pt=6  arith_type=Boolean  quantization=Truncate  overflow=Wrap  hdl_port=on  timing_constraint=None  locs_specified=off  LOCs={}  needs_fixed_name=off  show_param=off
      settings: xl_area=[0, 0, 0, 0, 0, 0, 0]
  seti_ct_sys_dram_ctrl_dimm1_Mem_Wr_Din : xbsIndex_r3/Gateway Out  output_type=Double  nbits=8  bin_pt=6  arith_type=Boolean  quantization=Truncate  overflow=Wrap  hdl_port=on  timing_constraint=None  locs_specified=off  LOCs={}  needs_fixed_name=off  show_param=off
      settings: xl_area=[0, 0, 0, 0, 0, 0, 0]
  sim_wrapper : Subsystem
  cmd_ack : Outport
  data_out : Outport  Port=2
  rd_tag : Outport  Port=3
  rd_valid : Outport  Port=4
  wires:
  force_rd_dout/1 -> data_out/1
  force_data_in/1 -> seti_ct_sys_dram_ctrl_dimm1_Mem_Wr_Din/1, sim_wrapper/3(data_in)
  convert_rd_ack/1 -> seti_ct_sys_dram_ctrl_dimm1_Mem_Rd_Ack/1, sim_wrapper/8(rd_ack)
  convert_cmd_valid/1 -> seti_ct_sys_dram_ctrl_dimm1_Mem_Cmd_Valid/1, sim_wrapper/7(cmd_valid)
  convert_cmd_tag/1 -> seti_ct_sys_dram_ctrl_dimm1_Mem_Cmd_Tag/1, sim_wrapper/6(cmd_tag)
  convert_rwn/1 -> seti_ct_sys_dram_ctrl_dimm1_Mem_Cmd_RNW/1, sim_wrapper/5(RWn)
  convert_wr_be/1 -> seti_ct_sys_dram_ctrl_dimm1_Mem_Wr_BE/1, sim_wrapper/4(wr_be)
  convert_data_in/1 -> force_data_in/1
  convert_address/1 -> seti_ct_sys_dram_ctrl_dimm1_Mem_Cmd_Address/1, sim_wrapper/2(address)
  convert_rst/1 -> seti_ct_sys_dram_ctrl_dimm1_Mem_Rst/1, sim_wrapper/1(rst)
  rd_ack/1 -> convert_rd_ack/1
  cmd_valid/1 -> convert_cmd_valid/1
  cmd_tag/1 -> convert_cmd_tag/1
  RWn/1 -> convert_rwn/1
  data_in/1 -> convert_data_in/1
  rst/1 -> convert_rst/1
  address/1 -> convert_address/1
  wr_be/1 -> convert_wr_be/1
  seti_ct_sys_dram_ctrl_dimm1_Mem_Rst/1 -> Terminator/1
  seti_ct_sys_dram_ctrl_dimm1_Mem_Cmd_Address/1 -> Terminator1/1
  seti_ct_sys_dram_ctrl_dimm1_Mem_Wr_Din/1 -> Terminator2/1
  seti_ct_sys_dram_ctrl_dimm1_Mem_Wr_BE/1 -> Terminator3/1
  seti_ct_sys_dram_ctrl_dimm1_Mem_Cmd_RNW/1 -> Terminator4/1
  seti_ct_sys_dram_ctrl_dimm1_Mem_Cmd_Tag/1 -> Terminator5/1
  seti_ct_sys_dram_ctrl_dimm1_Mem_Cmd_Valid/1 -> Terminator6/1
  seti_ct_sys_dram_ctrl_dimm1_Mem_Rd_Ack/1 -> Terminator7/1
  Constant/1 -> seti_ct_sys_dram_ctrl_dimm1_Mem_Cmd_Ack/1, seti_ct_sys_dram_ctrl_dimm1_Mem_Rd_Dout/1, seti_ct_sys_dram_ctrl_dimm1_Mem_Rd_Tag/1, seti_ct_sys_dram_ctrl_dimm1_Mem_Rd_Valid/1
  seti_ct_sys_dram_ctrl_dimm1_Mem_Cmd_Ack/1 -> Simulation Multiplexer/1
  Simulation Multiplexer/1 -> cmd_ack/1
  seti_ct_sys_dram_ctrl_dimm1_Mem_Rd_Dout/1 -> Simulation Multiplexer1/1
  Simulation Multiplexer1/1 -> force_rd_dout/1
  Simulation Multiplexer2/1 -> rd_tag/1
  Simulation Multiplexer3/1 -> rd_valid/1
  seti_ct_sys_dram_ctrl_dimm1_Mem_Rd_Tag/1 -> Simulation Multiplexer2/1
  seti_ct_sys_dram_ctrl_dimm1_Mem_Rd_Valid/1 -> Simulation Multiplexer3/1
  sim_wrapper/1(cmd_ack) -> Simulation Multiplexer/2
  sim_wrapper/2(data_out) -> Simulation Multiplexer1/2
  sim_wrapper/3(rd_tag) -> Simulation Multiplexer2/2
  sim_wrapper/4(rd_valid) -> Simulation Multiplexer3/2

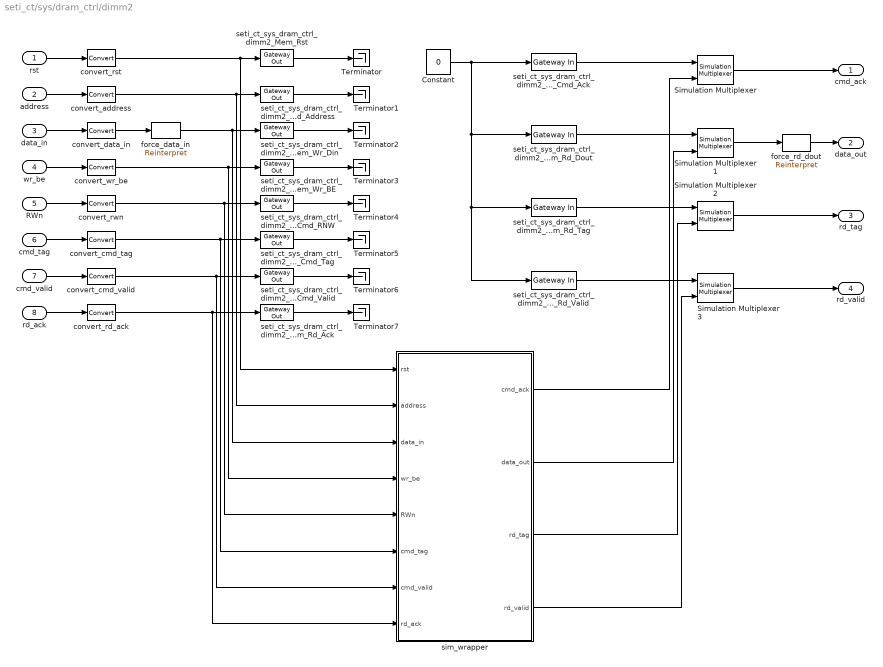
== system seti_ct/sys/dram_ctrl/dimm2 ==
  rst : Inport  Port=1  LatchInput=off
  address : Inport  Port=2  LatchInput=off
  data_in : Inport  Port=3  LatchInput=off
  wr_be : Inport  Port=4  LatchInput=off
  RWn : Inport  Port=5  LatchInput=off
  cmd_tag : Inport  Port=6  LatchInput=off
  cmd_valid : Inport  Port=7  LatchInput=off
  rd_ack : Inport  Port=8  LatchInput=off
  Constant : Constant  Value=0
  Simulation Multiplexer{,1..3} (4 alike) : xbsIndex_r3/Simulation Multiplexer  sim_sel=2  hw_sel=1
  Terminator{,1..7} (8 alike) : Terminator
  convert_address : xbsIndex_r3/Convert  arith_type=Unsigned  n_bits=32  bin_pt=0  quantization=Truncate  overflow=Wrap  latency=0  explicit_period=off  period=sample_period  dbl_ovrd=off  show_param=off  inserted_by_tool=off  pipeline=off
      settings: xl_area=[0, 0, 0, 0, 0, 0, 0]
  convert_cmd_tag : xbsIndex_r3/Convert  arith_type=Unsigned  n_bits=32  bin_pt=0  quantization=Truncate  overflow=Wrap  latency=0  explicit_period=off  period=1  dbl_ovrd=off  show_param=off  inserted_by_tool=off  pipeline=off
      settings: xl_area=[0, 0, 0, 0, 0, 0, 0]
  convert_cmd_valid : xbsIndex_r3/Convert  arith_type=Unsigned  n_bits=1  bin_pt=0  quantization=Truncate  overflow=Wrap  latency=0  explicit_period=off  period=1  dbl_ovrd=off  show_param=off  inserted_by_tool=off  pipeline=off
      settings: xl_area=[0, 0, 0, 0, 0, 0, 0]
  convert_data_in : xbsIndex_r3/Convert  arith_type=Unsigned  n_bits=144  bin_pt=0  quantization=Truncate  overflow=Wrap  latency=0  explicit_period=off  period=sample_period  dbl_ovrd=off  show_param=off  inserted_by_tool=off  pipeline=off
      settings: xl_area=[0, 0, 0, 0, 0, 0, 0]
  convert_rd_ack : xbsIndex_r3/Convert  arith_type=Unsigned  n_bits=1  bin_pt=0  quantization=Truncate  overflow=Wrap  latency=0  explicit_period=off  period=1  dbl_ovrd=off  show_param=off  inserted_by_tool=off  pipeline=off
      settings: xl_area=[0, 0, 0, 0, 0, 0, 0]
  convert_rst : xbsIndex_r3/Convert  arith_type=Unsigned  n_bits=1  bin_pt=0  quantization=Truncate  overflow=Wrap  latency=0  explicit_period=off  period=sample_period  dbl_ovrd=off  show_param=off  inserted_by_tool=off  pipeline=off
      settings: xl_area=[0, 0, 0, 0, 0, 0, 0]
  convert_rwn : xbsIndex_r3/Convert  arith_type=Unsigned  n_bits=1  bin_pt=0  quantization=Truncate  overflow=Wrap  latency=0  explicit_period=off  period=1  dbl_ovrd=off  show_param=off  inserted_by_tool=off  pipeline=off
      settings: xl_area=[0, 0, 0, 0, 0, 0, 0]
  convert_wr_be : xbsIndex_r3/Convert  arith_type=Unsigned  n_bits=18  bin_pt=0  quantization=Truncate  overflow=Wrap  latency=0  explicit_period=off  period=1  dbl_ovrd=off  show_param=off  inserted_by_tool=off  pipeline=off
      settings: xl_area=[0, 0, 0, 0, 0, 0, 0]
  force_data_in : xbsIndex_r3/Reinterpret  force_arith_type=on  arith_type=Unsigned  force_bin_pt=on  bin_pt=0  force_valid=on
  force_rd_dout : xbsIndex_r3/Reinterpret  force_arith_type=on  arith_type=Unsigned  force_bin_pt=on  bin_pt=0  force_valid=on
  seti_ct_sys_dram_ctrl_dimm2_Mem_Cmd_Ack : xbsIndex_r3/Gateway In  arith_type=Unsigned  n_bits=1  bin_pt=0  quantization=Truncate  overflow=Wrap  period=sample_period  timing_constraint=None  locs_specified=off  LOCs={}  needs_fixed_name=off  dbl_ovrd=off  show_param=off
      settings: xl_area=[0, 0, 0, 0, 0, 0, 0]
  seti_ct_sys_dram_ctrl_dimm2_Mem_Cmd_Address : xbsIndex_r3/Gateway Out  output_type=Double  nbits=8  bin_pt=6  arith_type=Boolean  quantization=Truncate  overflow=Wrap  hdl_port=on  timing_constraint=None  locs_specified=off  LOCs={}  needs_fixed_name=off  show_param=off
      settings: xl_area=[0, 0, 0, 0, 0, 0, 0]
  seti_ct_sys_dram_ctrl_dimm2_Mem_Cmd_RNW : xbsIndex_r3/Gateway Out  output_type=Double  nbits=8  bin_pt=6  arith_type=Boolean  quantization=Truncate  overflow=Wrap  hdl_port=on  timing_constraint=None  locs_specified=off  LOCs={}  needs_fixed_name=off  show_param=off
      settings: xl_area=[0, 0, 0, 0, 0, 0, 0]
  seti_ct_sys_dram_ctrl_dimm2_Mem_Cmd_Tag : xbsIndex_r3/Gateway Out  output_type=Double  nbits=8  bin_pt=6  arith_type=Boolean  quantization=Truncate  overflow=Wrap  hdl_port=on  timing_constraint=None  locs_specified=off  LOCs={}  needs_fixed_name=off  show_param=off
      settings: xl_area=[0, 0, 0, 0, 0, 0, 0]
  seti_ct_sys_dram_ctrl_dimm2_Mem_Cmd_Valid : xbsIndex_r3/Gateway Out  output_type=Double  nbits=8  bin_pt=6  arith_type=Boolean  quantization=Truncate  overflow=Wrap  hdl_port=on  timing_constraint=None  locs_specified=off  LOCs={}  needs_fixed_name=off  show_param=off
      settings: xl_area=[0, 0, 0, 0, 0, 0, 0]
  seti_ct_sys_dram_ctrl_dimm2_Mem_Rd_Ack : xbsIndex_r3/Gateway Out  output_type=Double  nbits=8  bin_pt=6  arith_type=Boolean  quantization=Truncate  overflow=Wrap  hdl_port=on  timing_constraint=None  locs_specified=off  LOCs={}  needs_fixed_name=off  show_param=off
      settings: xl_area=[0, 0, 0, 0, 0, 0, 0]
  seti_ct_sys_dram_ctrl_dimm2_Mem_Rd_Dout : xbsIndex_r3/Gateway In  arith_type=Unsigned  n_bits=144  bin_pt=0  quantization=Truncate  overflow=Wrap  period=sample_period  timing_constraint=None  locs_specified=off  LOCs={}  needs_fixed_name=off  dbl_ovrd=off  show_param=off
      settings: xl_area=[0, 0, 0, 0, 0, 0, 0]
  seti_ct_sys_dram_ctrl_dimm2_Mem_Rd_Tag : xbsIndex_r3/Gateway In  arith_type=Unsigned  n_bits=32  bin_pt=0  quantization=Truncate  overflow=Wrap  period=sample_period  timing_constraint=None  locs_specified=off  LOCs={}  needs_fixed_name=off  dbl_ovrd=off  show_param=off
      settings: xl_area=[0, 0, 0, 0, 0, 0, 0]
  seti_ct_sys_dram_ctrl_dimm2_Mem_Rd_Valid : xbsIndex_r3/Gateway In  arith_type=Unsigned  n_bits=1  bin_pt=0  quantization=Truncate  overflow=Wrap  period=sample_period  timing_constraint=None  locs_specified=off  LOCs={}  needs_fixed_name=off  dbl_ovrd=off  show_param=off
      settings: xl_area=[0, 0, 0, 0, 0, 0, 0]
  seti_ct_sys_dram_ctrl_dimm2_Mem_Rst : xbsIndex_r3/Gateway Out  output_type=Double  nbits=8  bin_pt=6  arith_type=Boolean  quantization=Truncate  overflow=Wrap  hdl_port=on  timing_constraint=None  locs_specified=off  LOCs={}  needs_fixed_name=off  show_param=off
      settings: xl_area=[0, 0, 0, 0, 0, 0, 0]
  seti_ct_sys_dram_ctrl_dimm2_Mem_Wr_BE : xbsIndex_r3/Gateway Out  output_type=Double  nbits=8  bin_pt=6  arith_type=Boolean  quantization=Truncate  overflow=Wrap  hdl_port=on  timing_constraint=None  locs_specified=off  LOCs={}  needs_fixed_name=off  show_param=off
      settings: xl_area=[0, 0, 0, 0, 0, 0, 0]
  seti_ct_sys_dram_ctrl_dimm2_Mem_Wr_Din : xbsIndex_r3/Gateway Out  output_type=Double  nbits=8  bin_pt=6  arith_type=Boolean  quantization=Truncate  overflow=Wrap  hdl_port=on  timing_constraint=None  locs_specified=off  LOCs={}  needs_fixed_name=off  show_param=off
      settings: xl_area=[0, 0, 0, 0, 0, 0, 0]
  sim_wrapper : Subsystem
  cmd_ack : Outport
  data_out : Outport  Port=2
  rd_tag : Outport  Port=3
  rd_valid : Outport  Port=4
  wires:
  force_rd_dout/1 -> data_out/1
  force_data_in/1 -> seti_ct_sys_dram_ctrl_dimm2_Mem_Wr_Din/1, sim_wrapper/3(data_in)
  convert_rd_ack/1 -> seti_ct_sys_dram_ctrl_dimm2_Mem_Rd_Ack/1, sim_wrapper/8(rd_ack)
  convert_cmd_valid/1 -> seti_ct_sys_dram_ctrl_dimm2_Mem_Cmd_Valid/1, sim_wrapper/7(cmd_valid)
  convert_cmd_tag/1 -> seti_ct_sys_dram_ctrl_dimm2_Mem_Cmd_Tag/1, sim_wrapper/6(cmd_tag)
  convert_rwn/1 -> seti_ct_sys_dram_ctrl_dimm2_Mem_Cmd_RNW/1, sim_wrapper/5(RWn)
  convert_wr_be/1 -> seti_ct_sys_dram_ctrl_dimm2_Mem_Wr_BE/1, sim_wrapper/4(wr_be)
  convert_data_in/1 -> force_data_in/1
  convert_address/1 -> seti_ct_sys_dram_ctrl_dimm2_Mem_Cmd_Address/1, sim_wrapper/2(address)
  convert_rst/1 -> seti_ct_sys_dram_ctrl_dimm2_Mem_Rst/1, sim_wrapper/1(rst)
  rd_ack/1 -> convert_rd_ack/1
  cmd_valid/1 -> convert_cmd_valid/1
  cmd_tag/1 -> convert_cmd_tag/1
  RWn/1 -> convert_rwn/1
  data_in/1 -> convert_data_in/1
  rst/1 -> convert_rst/1
  address/1 -> convert_address/1
  wr_be/1 -> convert_wr_be/1
  seti_ct_sys_dram_ctrl_dimm2_Mem_Rst/1 -> Terminator/1
  seti_ct_sys_dram_ctrl_dimm2_Mem_Cmd_Address/1 -> Terminator1/1
  seti_ct_sys_dram_ctrl_dimm2_Mem_Wr_Din/1 -> Terminator2/1
  seti_ct_sys_dram_ctrl_dimm2_Mem_Wr_BE/1 -> Terminator3/1
  seti_ct_sys_dram_ctrl_dimm2_Mem_Cmd_RNW/1 -> Terminator4/1
  seti_ct_sys_dram_ctrl_dimm2_Mem_Cmd_Tag/1 -> Terminator5/1
  seti_ct_sys_dram_ctrl_dimm2_Mem_Cmd_Valid/1 -> Terminator6/1
  seti_ct_sys_dram_ctrl_dimm2_Mem_Rd_Ack/1 -> Terminator7/1
  Constant/1 -> seti_ct_sys_dram_ctrl_dimm2_Mem_Cmd_Ack/1, seti_ct_sys_dram_ctrl_dimm2_Mem_Rd_Dout/1, seti_ct_sys_dram_ctrl_dimm2_Mem_Rd_Tag/1, seti_ct_sys_dram_ctrl_dimm2_Mem_Rd_Valid/1
  seti_ct_sys_dram_ctrl_dimm2_Mem_Cmd_Ack/1 -> Simulation Multiplexer/1
  Simulation Multiplexer/1 -> cmd_ack/1
  seti_ct_sys_dram_ctrl_dimm2_Mem_Rd_Dout/1 -> Simulation Multiplexer1/1
  Simulation Multiplexer1/1 -> force_rd_dout/1
  Simulation Multiplexer2/1 -> rd_tag/1
  Simulation Multiplexer3/1 -> rd_valid/1
  seti_ct_sys_dram_ctrl_dimm2_Mem_Rd_Tag/1 -> Simulation Multiplexer2/1
  seti_ct_sys_dram_ctrl_dimm2_Mem_Rd_Valid/1 -> Simulation Multiplexer3/1
  sim_wrapper/1(cmd_ack) -> Simulation Multiplexer/2
  sim_wrapper/2(data_out) -> Simulation Multiplexer1/2
  sim_wrapper/3(rd_tag) -> Simulation Multiplexer2/2
  sim_wrapper/4(rd_valid) -> Simulation Multiplexer3/2
